simulink model "BuckBoost"  (R2019b)
settings: Solver=VariableStepAuto  StartTime=0.0  StopTime=216/fs_boost  RelTol=1e-3
values from neighbouring files (symbols this model uses):
  fs = 1000e3    (= 1000000)    [PLECS_Perameters_Buck_Boost.m]
undefined symbols (not defined in the file or in its folder): fixed, plecs
libraries: powerlib_meascontrol x4, plecslib_extras2 x1
settings Model: Creator=jb  LastModifiedBy=jb
settings DataIOCC: ReturnWorkspaceOutputs=off
settings DebuggingCC: MaxConsecutiveZCsMsg=warning  IgnoredZcDiagnostic=none  SolverPrmCheckMsg=warning

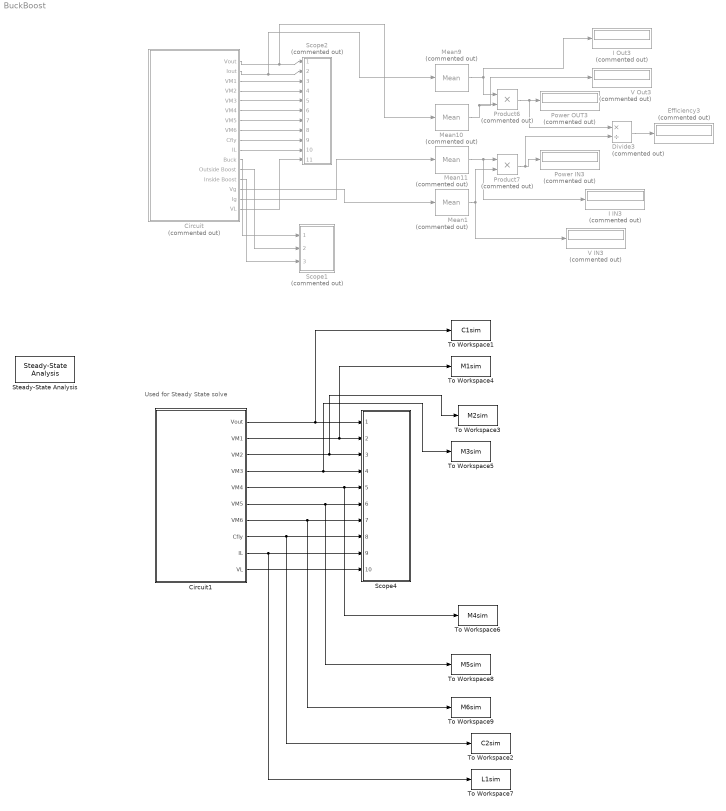
== system BuckBoost ==
  note: Used for Steady State solve
  Circuit : Subsystem  Commented=on  LoadFcn=plecs('sl', 200);  InitFcn=plecs('sl', 214);  StartFcn=plecs('sl', 208);  StopFcn=plecs('sl', 209);  mask(PlecsCircuit){PLECSData=<binary blob, 4652 chars, not shown>}
      mask prompts: PLECSData "PLECS Data (Do not delete or modify!)"
      mask init:
      | % PLACE CUSTOM INITIALIZATIONS ABOVE
      | % DO NOT REMOVE
      | plecs('sl', 215);
      | % DO NOT REMOVE
      settings: CopyFcn=plecs('sl', 203);  DeleteFcn=plecs('sl', 205);  UndoDeleteFcn=plecs('sl', 206);  PreSaveFcn=plecs('sl', 211);  PostSaveFcn=plecs('sl', 201);  NameChangeFcn=plecs('sl', 210);  DestroyFcn=plecs('sl', 207);  PreCopyFcn=plecs('sl', 216);  OpenFcn=plecs('sl', 202);  ErrorFcn=plerrorfcn
      mask Help: web(['file:///' fullfile(plecsdoc, 'creatingacircuit.html')])
      mask Display: disp('PLECS\nCircuit')
  Circuit1 : Subsystem  LoadFcn=plecs('sl', 200);  InitFcn=plecs('sl', 214);  StartFcn=plecs('sl', 208);  StopFcn=plecs('sl', 209);  mask(PlecsCircuit){PLECSData=<binary blob, 4104 chars, not shown>}
      mask prompts: PLECSData "PLECS Data (Do not delete or modify!)"
      mask init:
      | % PLACE CUSTOM INITIALIZATIONS ABOVE
      | % DO NOT REMOVE
      | plecs('sl', 215);
      | % DO NOT REMOVE
      settings: CopyFcn=plecs('sl', 203);  DeleteFcn=plecs('sl', 205);  UndoDeleteFcn=plecs('sl', 206);  PreSaveFcn=plecs('sl', 211);  PostSaveFcn=plecs('sl', 201);  NameChangeFcn=plecs('sl', 210);  DestroyFcn=plecs('sl', 207);  PreCopyFcn=plecs('sl', 216);  OpenFcn=plecs('sl', 202);  ErrorFcn=plerrorfcn
      mask Help: web(['file:///' fullfile(plecsdoc, 'creatingacircuit.html')])
      mask Display: disp('PLECS\nCircuit')
  Divide3 : Product  Commented=on  Inputs=*/
  Efficiency3 : Display  Commented=on
  I IN3 : Display  Commented=on
  I Out3 : Display  Commented=on
  Mean{1,9..11} (4 alike) : powerlib_meascontrol/Measurements/Mean  Commented=on  Freq=fs/10  Vinit=0  Ts=0
      settings: SourceProductName=Simscape Electrical
  Power IN3 : Display  Commented=on
  Power OUT3 : Display  Commented=on
  Product6 : Product  Commented=on
  Product7 : Product  Commented=on
  Scope1 : Subsystem  Commented=on  LoadFcn=plecs('sl', 300);  InitFcn=plecs('sl', 314);  StartFcn=plecs('sl', 308);  StopFcn=plecs('sl', 309);  mask{Settings=<binary blob, 1440 chars, not shown>}
      mask init:
      | plecs('sl', 315);
      settings: CopyFcn=plecs('sl', 303);  DeleteFcn=plecs('sl', 305);  UndoDeleteFcn=plecs('sl', 306);  PreSaveFcn=plecs('sl', 311);  NameChangeFcn=plecs('sl', 310);  DestroyFcn=plecs('sl', 307);  OpenFcn=plecs('sl', 302);  ErrorFcn=plerrorfcn
      mask Display: plot([0.1 0.9 0.9 0.1 0.1], [0.9 0.9 0.5 0.5 0.9])
  Scope2 : Subsystem  Commented=on  LoadFcn=plecs('sl', 300);  InitFcn=plecs('sl', 314);  StartFcn=plecs('sl', 308);  StopFcn=plecs('sl', 309);  mask{Settings=<binary blob, 2836 chars, not shown>}
      mask init:
      | plecs('sl', 315);
      settings: CopyFcn=plecs('sl', 303);  DeleteFcn=plecs('sl', 305);  UndoDeleteFcn=plecs('sl', 306);  PreSaveFcn=plecs('sl', 311);  NameChangeFcn=plecs('sl', 310);  DestroyFcn=plecs('sl', 307);  OpenFcn=plecs('sl', 302);  ErrorFcn=plerrorfcn
      mask Display: plot([0.1 0.9 0.9 0.1 0.1], [0.9 0.9 0.5 0.5 0.9])
  Scope4 : Subsystem  LoadFcn=plecs('sl', 300);  InitFcn=plecs('sl', 314);  StartFcn=plecs('sl', 308);  StopFcn=plecs('sl', 309);  mask{Settings=<binary blob, 2300 chars, not shown>}
      mask init:
      | plecs('sl', 315);
      settings: CopyFcn=plecs('sl', 303);  DeleteFcn=plecs('sl', 305);  UndoDeleteFcn=plecs('sl', 306);  PreSaveFcn=plecs('sl', 311);  NameChangeFcn=plecs('sl', 310);  DestroyFcn=plecs('sl', 307);  OpenFcn=plecs('sl', 302);  ErrorFcn=plerrorfcn
      mask Display: plot([0.1 0.9 0.9 0.1 0.1], [0.9 0.9 0.5 0.5 0.9])
  Steady-State Analysis : plecslib_extras2/Analysis Tools/Steady-State Analysis  Period=fixed  TriggerType=rising  TimeSpan=1e-5  TStart=0  MaxIter=20  Tolerance=1e-6  Display=iteration  HideScopes=off  HiddenStates=error  FinalStateName=xSteadyState  NCycles=3  JPert=1e-4  JacobianCalculation=fast  NInitCycles=0
      settings: SourceProductName=PLECS Extras
  To Workspace1 : ToWorkspace  VariableName=C1sim  SaveFormat=Timeseries  SampleTime=-1
  To Workspace2 : ToWorkspace  VariableName=C2sim  SaveFormat=Timeseries  SampleTime=-1
  To Workspace3 : ToWorkspace  VariableName=M2sim  SaveFormat=Timeseries  SampleTime=-1
  To Workspace4 : ToWorkspace  VariableName=M1sim  SaveFormat=Timeseries  SampleTime=-1
  To Workspace5 : ToWorkspace  VariableName=M3sim  SaveFormat=Timeseries  SampleTime=-1
  To Workspace6 : ToWorkspace  VariableName=M4sim  SaveFormat=Timeseries  SampleTime=-1
  To Workspace7 : ToWorkspace  VariableName=L1sim  SaveFormat=Timeseries  SampleTime=-1
  To Workspace8 : ToWorkspace  VariableName=M5sim  SaveFormat=Timeseries  SampleTime=-1
  To Workspace9 : ToWorkspace  VariableName=M6sim  SaveFormat=Timeseries  SampleTime=-1
  V IN3 : Display  Commented=on
  V Out3 : Display  Commented=on
  wires:
  Circuit/1(Vout) -> Mean10/1, Scope2/1(1)
  Circuit/2(Iout) -> Mean9/1, Scope2/2(2)
  Circuit/3(VM1) -> Scope2/3(3)
  Circuit/4(VM2) -> Scope2/4(4)
  Circuit/5(VM3) -> Scope2/5(5)
  Circuit/6(VM4) -> Scope2/6(6)
  Circuit/7(VM5) -> Scope2/7(7)
  Circuit/8(VM6) -> Scope2/8(8)
  Circuit/9(Cfly) -> Scope2/9(9)
  Circuit/10(IL) -> Scope2/10(10)
  Circuit/11(Buck) -> Scope1/1(1)
  Circuit/12(Outside Boost) -> Scope1/2(2)
  Circuit/13(Inside Boost) -> Scope1/3(3)
  Mean1/1 -> V IN3/1, Product7/2
  Divide3/1 -> Efficiency3/1
  Mean9/1 -> Product6/1, I Out3/1
  Product7/1 -> Divide3/2, Power IN3/1
  Mean11/1 -> I IN3/1, Product7/1
  Product6/1 -> Divide3/1, Power OUT3/1
  Mean10/1 -> V Out3/1, Product6/2
  Circuit/14(Vg) -> Mean1/1
  Circuit/15(Ig) -> Mean11/1
  Circuit/16(VL) -> Scope2/11(11)
  Circuit1/1(Vout) -> To Workspace1/1, Scope4/1(1)
  Circuit1/2(VM1) -> To Workspace4/1, Scope4/2(2)
  Circuit1/3(VM2) -> To Workspace3/1, Scope4/3(3)
  Circuit1/4(VM3) -> To Workspace5/1, Scope4/4(4)
  Circuit1/5(VM4) -> To Workspace6/1, Scope4/5(5)
  Circuit1/6(VM5) -> To Workspace8/1, Scope4/6(6)
  Circuit1/7(VM6) -> To Workspace9/1, Scope4/7(7)
  Circuit1/8(Cfly) -> To Workspace2/1, Scope4/8(8)
  Circuit1/9(IL) -> To Workspace7/1, Scope4/9(9)
  Circuit1/10(VL) -> Scope4/10(10)

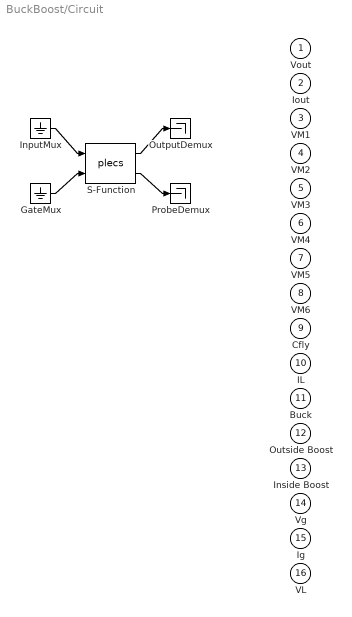
== system BuckBoost/Circuit ==
  " GateMux " : Ground
  " InputMux " : Ground
  " OutputDemux " : Terminator
  " ProbeDemux " : Terminator
  " S-Function " : S-Function  FunctionName=plecs  SFunctionDeploymentMode=off  EnableBusSupport=off
  Vout : Outport  PortDimensions=1
  Iout : Outport  Port=2  PortDimensions=1
  VM1 : Outport  Port=3  PortDimensions=1
  VM2 : Outport  Port=4  PortDimensions=1
  VM3 : Outport  Port=5  PortDimensions=1
  VM4 : Outport  Port=6  PortDimensions=1
  VM5 : Outport  Port=7  PortDimensions=1
  VM6 : Outport  Port=8  PortDimensions=1
  Cfly : Outport  Port=9  PortDimensions=1
  IL : Outport  Port=10  PortDimensions=1
  Buck : Outport  Port=11  PortDimensions=2
  Outside Boost : Outport  Port=12  PortDimensions=2
  Inside Boost : Outport  Port=13  PortDimensions=2
  Vg : Outport  Port=14  PortDimensions=1
  Ig : Outport  Port=15  PortDimensions=1
  VL : Outport  Port=16  PortDimensions=1
  wires:
  " InputMux "/1 -> " S-Function "/1
  " GateMux "/1 -> " S-Function "/2
  " S-Function "/1 -> " OutputDemux "/1
  " S-Function "/2 -> " ProbeDemux "/1

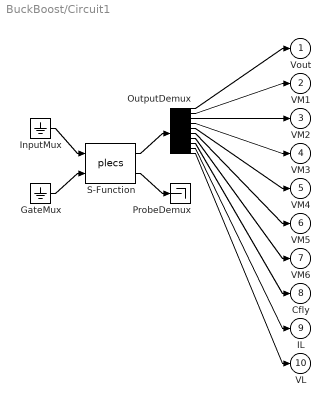
== system BuckBoost/Circuit1 ==
  " GateMux " : Ground
  " InputMux " : Ground
  " OutputDemux " : Demux  Outputs=[ 1 1 1 1 1 1 1 1 1 1 ]
  " ProbeDemux " : Terminator
  " S-Function " : S-Function  FunctionName=plecs  SFunctionDeploymentMode=off  EnableBusSupport=off
  Vout : Outport  PortDimensions=1
  VM1 : Outport  Port=2  PortDimensions=1
  VM2 : Outport  Port=3  PortDimensions=1
  VM3 : Outport  Port=4  PortDimensions=1
  VM4 : Outport  Port=5  PortDimensions=1
  VM5 : Outport  Port=6  PortDimensions=1
  VM6 : Outport  Port=7  PortDimensions=1
  Cfly : Outport  Port=8  PortDimensions=1
  IL : Outport  Port=9  PortDimensions=1
  VL : Outport  Port=10  PortDimensions=1
  wires:
  " InputMux "/1 -> " S-Function "/1
  " GateMux "/1 -> " S-Function "/2
  " S-Function "/1 -> " OutputDemux "/1
  " S-Function "/2 -> " ProbeDemux "/1
  " OutputDemux "/1 -> Vout/1
  " OutputDemux "/2 -> VM1/1
  " OutputDemux "/3 -> VM2/1
  " OutputDemux "/4 -> VM3/1
  " OutputDemux "/5 -> VM4/1
  " OutputDemux "/6 -> VM5/1
  " OutputDemux "/7 -> VM6/1
  " OutputDemux "/8 -> Cfly/1
  " OutputDemux "/9 -> IL/1
  " OutputDemux "/10 -> VL/1

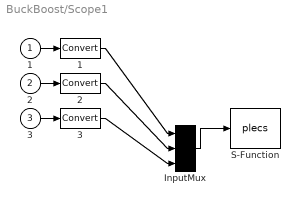
== system BuckBoost/Scope1 ==
  1 : Inport
  2 : Inport  Port=2
  3 : Inport  Port=3
  " 1 " : DataTypeConversion  SaturateOnIntegerOverflow=on  RndMeth=Zero
  " 2 " : DataTypeConversion  SaturateOnIntegerOverflow=on  RndMeth=Zero
  " 3 " : DataTypeConversion  SaturateOnIntegerOverflow=on  RndMeth=Zero
  " InputMux " : Mux  Inputs=3
  " S-Function " : S-Function  FunctionName=plecs  SFunctionDeploymentMode=off  EnableBusSupport=off
  wires:
  " InputMux "/1 -> " S-Function "/1
  1/1 -> " 1 "/1
  " 1 "/1 -> " InputMux "/1
  2/1 -> " 2 "/1
  " 2 "/1 -> " InputMux "/2
  3/1 -> " 3 "/1
  " 3 "/1 -> " InputMux "/3

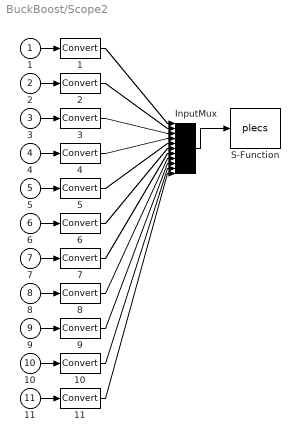
== system BuckBoost/Scope2 ==
  1 : Inport
  2 : Inport  Port=2
  3 : Inport  Port=3
  4 : Inport  Port=4
  5 : Inport  Port=5
  6 : Inport  Port=6
  7 : Inport  Port=7
  8 : Inport  Port=8
  9 : Inport  Port=9
  10 : Inport  Port=10
  11 : Inport  Port=11
  " 1 " : DataTypeConversion  SaturateOnIntegerOverflow=on  RndMeth=Zero
  " 10 " : DataTypeConversion  SaturateOnIntegerOverflow=on  RndMeth=Zero
  " 11 " : DataTypeConversion  SaturateOnIntegerOverflow=on  RndMeth=Zero
  " 2 " : DataTypeConversion  SaturateOnIntegerOverflow=on  RndMeth=Zero
  " 3 " : DataTypeConversion  SaturateOnIntegerOverflow=on  RndMeth=Zero
  " 4 " : DataTypeConversion  SaturateOnIntegerOverflow=on  RndMeth=Zero
  " 5 " : DataTypeConversion  SaturateOnIntegerOverflow=on  RndMeth=Zero
  " 6 " : DataTypeConversion  SaturateOnIntegerOverflow=on  RndMeth=Zero
  " 7 " : DataTypeConversion  SaturateOnIntegerOverflow=on  RndMeth=Zero
  " 8 " : DataTypeConversion  SaturateOnIntegerOverflow=on  RndMeth=Zero
  " 9 " : DataTypeConversion  SaturateOnIntegerOverflow=on  RndMeth=Zero
  " InputMux " : Mux  Inputs=11
  " S-Function " : S-Function  FunctionName=plecs  SFunctionDeploymentMode=off  EnableBusSupport=off
  wires:
  " InputMux "/1 -> " S-Function "/1
  1/1 -> " 1 "/1
  " 1 "/1 -> " InputMux "/1
  2/1 -> " 2 "/1
  " 2 "/1 -> " InputMux "/2
  3/1 -> " 3 "/1
  " 3 "/1 -> " InputMux "/3
  4/1 -> " 4 "/1
  " 4 "/1 -> " InputMux "/4
  5/1 -> " 5 "/1
  " 5 "/1 -> " InputMux "/5
  6/1 -> " 6 "/1
  " 6 "/1 -> " InputMux "/6
  7/1 -> " 7 "/1
  " 7 "/1 -> " InputMux "/7
  8/1 -> " 8 "/1
  " 8 "/1 -> " InputMux "/8
  9/1 -> " 9 "/1
  " 9 "/1 -> " InputMux "/9
  10/1 -> " 10 "/1
  " 10 "/1 -> " InputMux "/10
  11/1 -> " 11 "/1
  " 11 "/1 -> " InputMux "/11

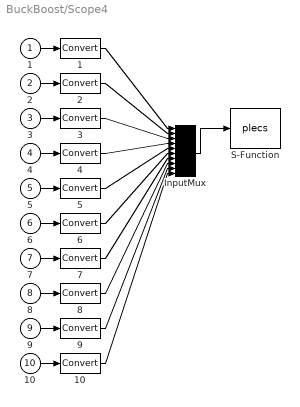
== system BuckBoost/Scope4 ==
  1 : Inport
  2 : Inport  Port=2
  3 : Inport  Port=3
  4 : Inport  Port=4
  5 : Inport  Port=5
  6 : Inport  Port=6
  7 : Inport  Port=7
  8 : Inport  Port=8
  9 : Inport  Port=9
  10 : Inport  Port=10
  " 1 " : DataTypeConversion  SaturateOnIntegerOverflow=on  RndMeth=Zero
  " 10 " : DataTypeConversion  SaturateOnIntegerOverflow=on  RndMeth=Zero
  " 2 " : DataTypeConversion  SaturateOnIntegerOverflow=on  RndMeth=Zero
  " 3 " : DataTypeConversion  SaturateOnIntegerOverflow=on  RndMeth=Zero
  " 4 " : DataTypeConversion  SaturateOnIntegerOverflow=on  RndMeth=Zero
  " 5 " : DataTypeConversion  SaturateOnIntegerOverflow=on  RndMeth=Zero
  " 6 " : DataTypeConversion  SaturateOnIntegerOverflow=on  RndMeth=Zero
  " 7 " : DataTypeConversion  SaturateOnIntegerOverflow=on  RndMeth=Zero
  " 8 " : DataTypeConversion  SaturateOnIntegerOverflow=on  RndMeth=Zero
  " 9 " : DataTypeConversion  SaturateOnIntegerOverflow=on  RndMeth=Zero
  " InputMux " : Mux  Inputs=10
  " S-Function " : S-Function  FunctionName=plecs  SFunctionDeploymentMode=off  EnableBusSupport=off
  wires:
  " InputMux "/1 -> " S-Function "/1
  1/1 -> " 1 "/1
  " 1 "/1 -> " InputMux "/1
  2/1 -> " 2 "/1
  " 2 "/1 -> " InputMux "/2
  3/1 -> " 3 "/1
  " 3 "/1 -> " InputMux "/3
  4/1 -> " 4 "/1
  " 4 "/1 -> " InputMux "/4
  5/1 -> " 5 "/1
  " 5 "/1 -> " InputMux "/5
  6/1 -> " 6 "/1
  " 6 "/1 -> " InputMux "/6
  7/1 -> " 7 "/1
  " 7 "/1 -> " InputMux "/7
  8/1 -> " 8 "/1
  " 8 "/1 -> " InputMux "/8
  9/1 -> " 9 "/1
  " 9 "/1 -> " InputMux "/9
  10/1 -> " 10 "/1
  " 10 "/1 -> " InputMux "/10
